simulink subsystem "no_filter"  (R2024b)
settings: Solver=VariableStepAuto  StartTime=0.0  StopTime=10.0  RelTol=1e-3
undefined symbols (not defined in the file or in its folder): airdata, GROUND_LEVEL, use_custom_atm
libraries: simulink x1
settings Model: Creator=yevge  LastModifiedBy=Aiden Gaydos

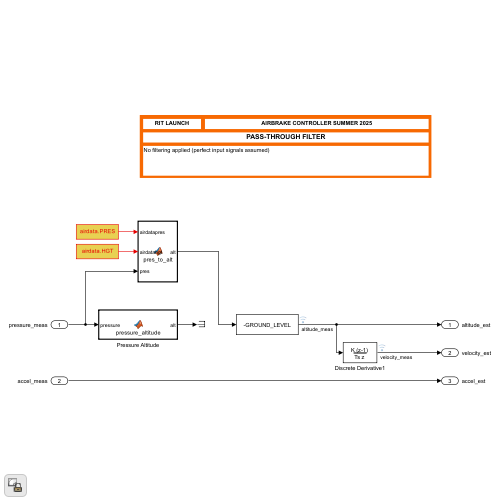
[thumbnail: Simulink's stored preview of the top-level diagram]
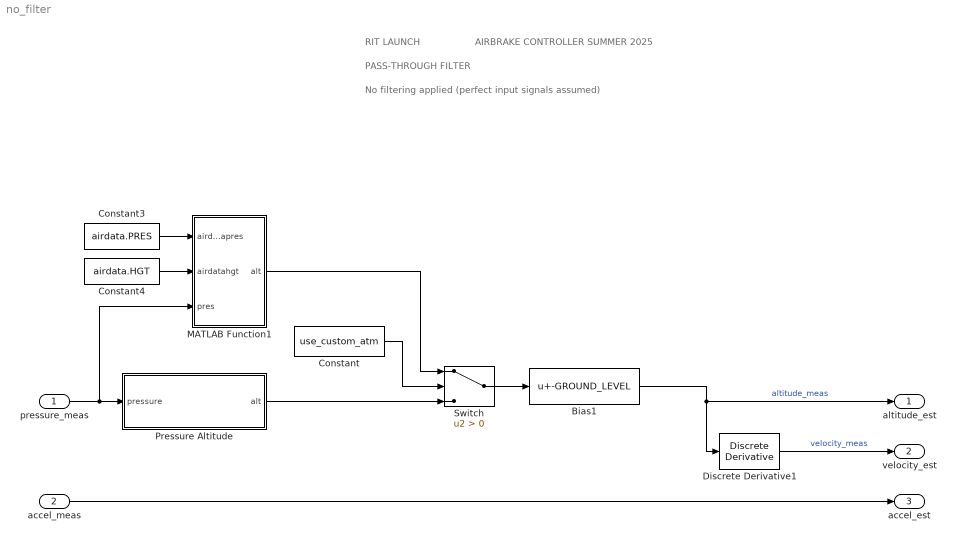
== system no_filter ==
  note: No filtering applied (perfect input signals assumed)
  note: PASS-THROUGH FILTER
  note: RIT LAUNCH
  note: AIRBRAKE CONTROLLER SUMMER 2025
  pressure_meas : Inport  Unit=Pa  PortDimensions=1
  accel_meas : Inport  Port=2  Unit=m/s^2  PortDimensions=1
  Bias1 : Bias  Bias=-GROUND_LEVEL  SaturateOnIntegerOverflow=off
  Constant : Constant  Value=use_custom_atm
  Constant3 : Constant  Value=airdata.PRES
  Constant4 : Constant  Value=airdata.HGT
  Discrete Derivative1 : simulink/Discrete/Discrete Derivative  gainval=1.0  ICPrevScaledInput=0.0  OutMin=[]  OutMax=[]  OutDataType=fixdt(1, 16)  OutScaling=2^-10  DoSatur=off
  MATLAB Function1 : MATLAB Function  TreatAsAtomicUnit=on
  Pressure Altitude : MATLAB Function  TreatAsAtomicUnit=on
  Switch : Switch  Criteria=u2 > Threshold  SaturateOnIntegerOverflow=off  InputSameDT=off
  altitude_est : Outport  Unit=m  PortDimensions=1
  velocity_est : Outport  Port=2  Unit=m/s  PortDimensions=1
  accel_est : Outport  Port=3  Unit=m/s^2  PortDimensions=1
  wires:
  pressure_meas/1 -> Pressure Altitude/1(pressure), MATLAB Function1/3(pres)
  Bias1/1 -> Discrete Derivative1/1, altitude_est/1  "altitude_meas"
  Discrete Derivative1/1 -> velocity_est/1  "velocity_meas"
  accel_meas/1 -> accel_est/1
  Constant3/1 -> MATLAB Function1/1(airdatapres)
  Constant4/1 -> MATLAB Function1/2(airdatahgt)
  Switch/1 -> Bias1/1
  Pressure Altitude/1(alt) -> Switch/3
  MATLAB Function1/1(alt) -> Switch/1
  Constant/1 -> Switch/2

== matlab function no_filter/Pressure Altitude ==
  data: pressure input; alt output
function alt = pressure_altitude(pressure)
    alt = (1 - (pressure ./ 101325).^(0.190284)) .* 145366.45 * 0.3048;
end

== matlab function no_filter/MATLAB Function1 ==
  data: airdatapres input; airdatahgt input; pres input; alt output
function alt = pres_to_alt(airdatapres,airdatahgt,pres)
    alt = double(interp1(airdatapres,airdatahgt,pres,"linear","extrap"));
end
